simulink model "inverted_pendulum_2018b"  (R2018b)
settings: Solver=VariableStepAuto  StartTime=0.0  StopTime=double(Tsim)  RelTol=1e-3
InitFcn:
  | x0 = [0.0, 0, pi, 0.2];
  | measurementNoiseVariance = 1e-5 * [1, 1, 1, 1];
  | dt = 1e-3;
  | Tsim = 3;
settings Model: Creator=ka59symi  LastModifiedBy=ka59symi
settings DataIOCC: ReturnWorkspaceOutputs=on
settings DebuggingCC: UnconnectedInputMsg=none  UnconnectedOutputMsg=none  UnconnectedLineMsg=none
settings ModelReferenceCC: EnableRefExpFcnMdlSchedulingChecks=off
settings RTWCC: Description=Generic Real-Time Target

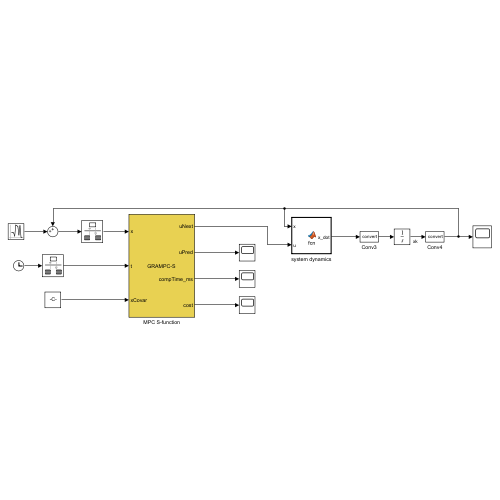
[thumbnail: Simulink's stored preview of the top-level diagram]
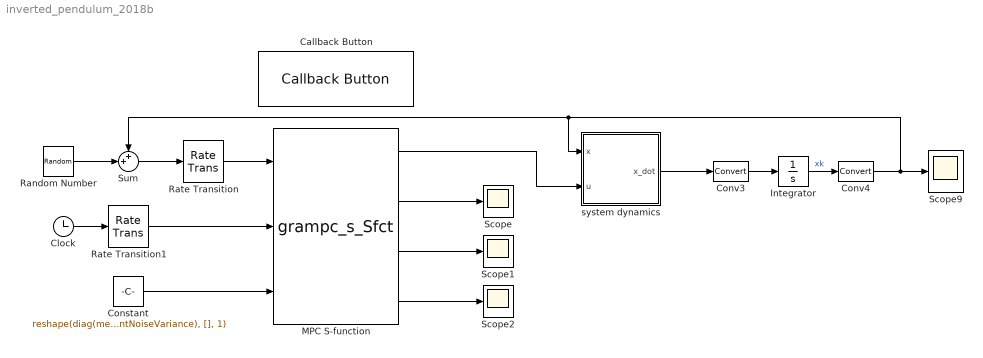
== system inverted_pendulum_2018b ==
  Callback Button : CallbackButton  WebBlockId=1  PressDelay=500  RepeatInterval=0  ButtonText=Click to compile S-function
      settings: ClickFcn=|
      | clc;
      | clear all;
      | 
      | path_to_grampc = fileparts(fileparts(cd));
      | 
      | probfct_inc = fullfile(cd, 'inverted_pendulum_problem_description.hpp');
      | probfct_src = fullfile(cd, 'inverted_pendulum_problem_description.cpp');
      | s_function  = fullfile(cd, 'grampc_s_Sfct.cpp');
      | 
      | addpath(fullfile(path_to_grampc, 'matlab'));
      | 
      | make_Sfunction(path_to_grampc, probfct_inc, probfct_src, s_function);
  Clock : Clock
  Constant : Constant  Value=reshape(diag(measurementNoiseVariance), [], 1)  VectorParams1D=off
  Conv3 : DataTypeConversion
  Conv4 : DataTypeConversion
  Integrator : Integrator  InitialCondition=x0
  MPC S-function : S-Function  FunctionName=grampc_s_Sfct  SFunctionDeploymentMode=off  EnableBusSupport=off
      mask Display:
      | port_label('input',1,'x')
      | port_label('input',2,'t')
      | port_label('input',3,'xCovar')
      | 
      | port_label('output',1,'uNext')
      | port_label('output',2,'uPred')
      | port_label('output',3,'compTime_ms')
      | port_label('output',4,'cost')
      | 
      | disp('GRAMPC-S')
  Random Number : RandomNumber  Mean=zeros(4,1)  Variance=measurementNoiseVariance  SampleTime=dt
  Rate Transition : RateTransition  OutPortSampleTime=dt
  Rate Transition1 : RateTransition  OutPortSampleTime=dt
  Scope{,1..2,9} (4 alike) : Scope
  Sum : Sum  Inputs=++|
  system dynamics : MATLAB Function  TreatAsAtomicUnit=on
  wires:
  Rate Transition/1 -> MPC S-function/1
  Random Number/1 -> Sum/2
  MPC S-function/3 -> Scope1/1
  MPC S-function/4 -> Scope2/1
  Sum/1 -> Rate Transition/1
  MPC S-function/2 -> Scope/1
  MPC S-function/1 -> system dynamics/2(u)
  Clock/1 -> Rate Transition1/1
  Integrator/1 -> Conv4/1  "xk"
  Constant/1 -> MPC S-function/3
  system dynamics/1(x_dot) -> Conv3/1
  Rate Transition1/1 -> MPC S-function/2
  Conv4/1 -> system dynamics/1(x), Sum/1, Scope9/1
  Conv3/1 -> Integrator/1

== matlab function inverted_pendulum_2018b/system dynamics ==
  data: x input; u input; x_dot output
function x_dot = fcn(x, u)
    x_dot = zeros(1, 4);

    x_dot(1) = x(2);
    x_dot(2) = u(1);
    x_dot(3) = x(4);
    x_dot(4) = -(2e-3*x(4)+0.2*(0.15*u(1)*cos(x(3))+0.15*9.81*sin(x(3))))/(1.3e-3+(0.2*0.2)*0.15);
end
